simulink model "lab3_model_2"  (R2015a)
settings: Solver=ode45  StartTime=0.0  StopTime=10.0  RelTol=1e-3
values from neighbouring files (symbols this model uses):
  A = 1    [script1.m]
undefined symbols (not defined in the file or in its folder): AP, B, BP, C, CP, WPC
settings Model: Creator=bb  LastModifiedBy=bb

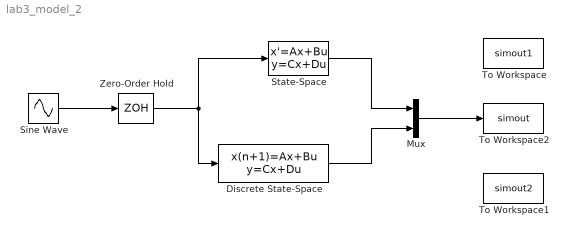
== system lab3_model_2 ==
  Discrete State-Space : DiscreteStateSpace  A=AP  B=BP  C=CP  D=[0;0]  X0=WPC
  Mux : Mux  Inputs=2
  Sine Wave : Sin  SampleTime=0
  State-Space : StateSpace  A=A  B=B  C=C  D=[0;0]  X0=WPC
  To Workspace : ToWorkspace  VariableName=simout1  SampleTime=-1
  To Workspace1 : ToWorkspace  VariableName=simout2  SaveFormat=Timeseries  SampleTime=-1
  To Workspace2 : ToWorkspace  VariableName=simout  SampleTime=-1
  Zero-Order Hold : ZeroOrderHold
  wires:
  Zero-Order Hold/1 -> State-Space/1, Discrete State-Space/1
  Sine Wave/1 -> Zero-Order Hold/1
  State-Space/1 -> Mux/1
  Discrete State-Space/1 -> Mux/2
  Mux/1 -> To Workspace2/1
